simulink model "slam"  (R2018a)
settings: Solver=VariableStepAuto  StartTime=0.0  StopTime=25  RelTol=1e-3
model workspace (MAT data in the model file):
  SL_ROS_VariableLengthArrays_MaxSizes.CommonInfo.ArrayTruncateAction = 'EmitWarning'
  SL_ROS_VariableLengthArrays_MaxSizes.MsgTypeMap = containers.Map
  SL_ROS_VariableLengthArrays_MaxSizes.MsgTypeMap.serialization.keys = {'sensor_msgs/LaserScan'}
  SL_ROS_VariableLengthArrays_MaxSizes.MsgTypeMap.serialization.values{1}(1).PropertyName = 'Intensities'
  SL_ROS_VariableLengthArrays_MaxSizes.MsgTypeMap.serialization.values{1}(1).DataType = 'single'
  SL_ROS_VariableLengthArrays_MaxSizes.MsgTypeMap.serialization.values{1}(1).MaxLength = 360
  SL_ROS_VariableLengthArrays_MaxSizes.MsgTypeMap.serialization.values{1}(2).PropertyName = 'Ranges'
  SL_ROS_VariableLengthArrays_MaxSizes.MsgTypeMap.serialization.values{1}(2).DataType = 'single'
  SL_ROS_VariableLengthArrays_MaxSizes.MsgTypeMap.serialization.values{1}(2).MaxLength = 360
  SL_ROS_VariableLengthArrays_MaxSizes.MsgTypeMap.serialization.uniformity = 0
  SL_ROS_VariableLengthArrays_MaxSizes.MsgTypeMap.serialization.keyType = 'char'
  SL_ROS_VariableLengthArrays_MaxSizes.MsgTypeMap.serialization.valueType = 'any'
undefined symbols (not defined in the file or in its folder): Angular, Linear
libraries: robotlib x6, simulink x1
settings Model: EnablePacing=on  Creator=gabriele  LastModifiedBy=gabriele

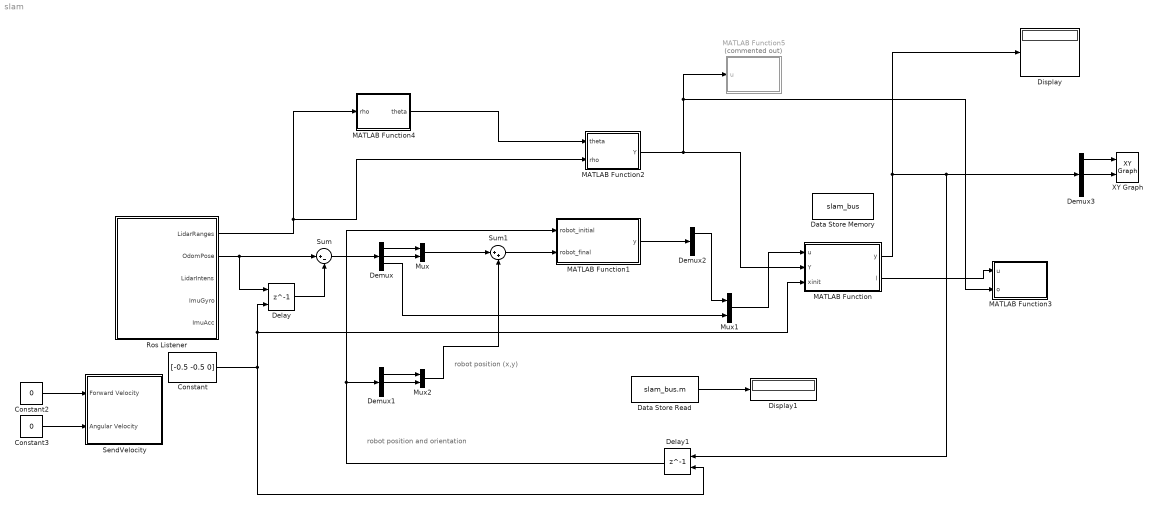
== system slam ==
  note: robot position
      | and orientation
  note: robot position (x,y)
  Constant : Constant  Value=[-0.5 -0.5 0]
  Constant2 : Constant  Value=0
  Constant3 : Constant  Value=0
  Data Store Memory : DataStoreMemory  DataStoreName=slam_bus  ReadBeforeWriteMsg=warning  WriteAfterWriteMsg=warning  WriteAfterReadMsg=warning  ShowAdditionalParam=off  OutDataTypeStr=Bus: slam_bus_t
  Data Store Read : DataStoreRead  DataStoreName=slam_bus  DataStoreElements=slam_bus.m
  Delay : Delay  DelayLength=1  InitialConditionSource=Input port  InitialCondition=[-0.5 -0.5 0]
      settings: InputPortMap=u0,p4
  Delay1 : Delay  DelayLength=1  InitialConditionSource=Input port  InitialCondition=zeros(3,1)
      settings: InputPortMap=u0,p4
  Demux : Demux  Outputs=3
  Demux1 : Demux  Outputs=3
  Demux2 : Demux  Outputs=2
  Demux3 : Demux  Outputs=3
  Display : Display
  Display1 : Display
  MATLAB Function : MATLAB Function  TreatAsAtomicUnit=on  mask{q=[0.1;0.1], s=[0.1;0.1]}
      mask prompts: q "Odometry Gaussian Noise"; s "Lidar Gaussian Noise"
  MATLAB Function1 : MATLAB Function  TreatAsAtomicUnit=on
  MATLAB Function2 : MATLAB Function  TreatAsAtomicUnit=on
  MATLAB Function3 : MATLAB Function  TreatAsAtomicUnit=on
  MATLAB Function4 : MATLAB Function  TreatAsAtomicUnit=on
  MATLAB Function5 : MATLAB Function  Commented=on  TreatAsAtomicUnit=on
  Mux : Mux  Inputs=2
  Mux1 : Mux  Inputs=2
  Mux2 : Mux  Inputs=2
  Ros Listener : Subsystem
  SendVelocity : Subsystem
  Sum : Sum  Inputs=|+-
  Sum1 : Sum  Inputs=|++
  XY Graph : simulink/Sinks/XY Graph  xmin=-1  xmax=1  ymin=-1  ymax=1  st=-1
  wires:
  Demux3/2 -> XY Graph/2
  Sum/1 -> Demux/1
  Ros Listener/2(OdomPose) -> Delay/1, Sum/1
  Delay1/1 -> Demux1/1, MATLAB Function1/1(robot_initial)
  Mux1/1 -> MATLAB Function/1(u)
  Delay/1 -> Sum/2
  MATLAB Function2/1(Y) -> MATLAB Function3/2(o), MATLAB Function5/1(u), MATLAB Function/2(Y)
  Mux/1 -> Sum1/1
  MATLAB Function/1(y) -> Display/1, Delay1/1, Demux3/1
  Demux/2 -> Mux/2
  Demux3/1 -> XY Graph/1
  Demux1/2 -> Mux2/2
  MATLAB Function1/1(y) -> Demux2/1
  Demux/1 -> Mux/1
  Mux2/1 -> Sum1/2
  Sum1/1 -> MATLAB Function1/2(robot_final)
  Demux1/1 -> Mux2/1
  Constant3/1 -> SendVelocity/2(Angular Velocity)
  Constant2/1 -> SendVelocity/1(Forward Velocity)
  Demux/3 -> Mux1/2
  Demux2/1 -> Mux1/1
  Ros Listener/1(LidarRanges) -> MATLAB Function2/2(rho), MATLAB Function4/1(rho)
  MATLAB Function4/1(theta) -> MATLAB Function2/1(theta)
  MATLAB Function/2(l) -> MATLAB Function3/1(u)
  Constant/1 -> Delay1/2, MATLAB Function/3(xinit), Delay/2
  Data Store Read/1 -> Display1/1

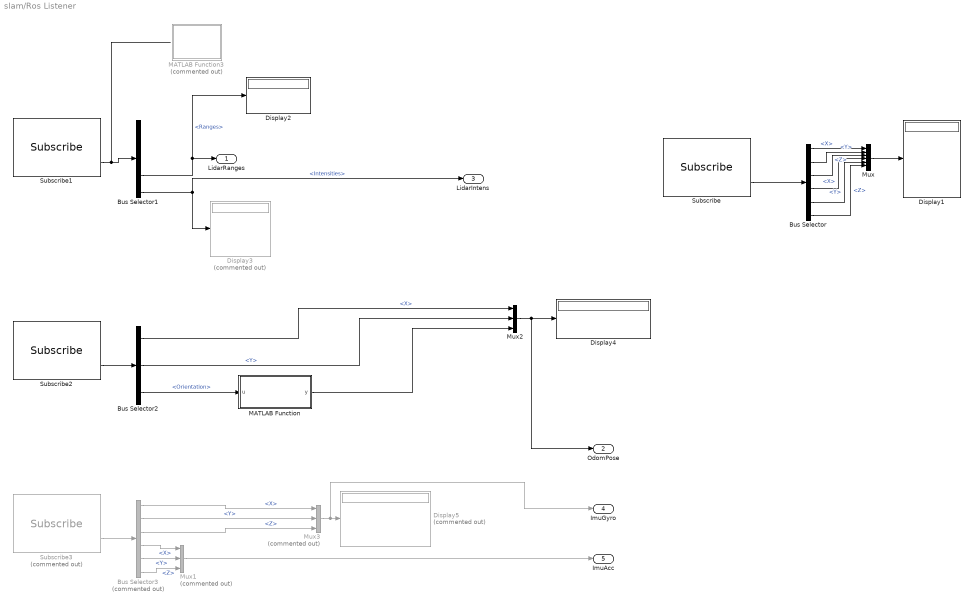
== system slam/Ros Listener ==
  Bus Selector : BusSelector  OutputSignals=Linear.X,Linear.Y,Linear.Z,Angular.X,Angular.Y,Angular.Z
  Bus Selector1 : BusSelector  OutputSignals=AngleMin,AngleMax,AngleIncrement,Ranges,Intensities
  Bus Selector2 : BusSelector  OutputSignals=Pose.Pose.Position.X,Pose.Pose.Position.Y,Pose.Pose.Orientation
  Bus Selector3 : BusSelector  Commented=on  OutputSignals=AngularVelocity.X,AngularVelocity.Y,AngularVelocity.Z,LinearAcceleration.X,LinearAcceleration.Y,LinearAcceleration.Z
  Display1 : Display
  Display2 : Display
  Display3 : Display  Commented=on
  Display4 : Display
  Display5 : Display  Commented=on
  MATLAB Function : MATLAB Function  TreatAsAtomicUnit=on
  MATLAB Function3 : MATLAB Function  Commented=on  TreatAsAtomicUnit=on
  Mux : Mux  Inputs=6
  Mux1 : Mux  Commented=on  Inputs=3
  Mux2 : Mux  Inputs=3
  Mux3 : Mux  Commented=on  Inputs=3
  Subscribe : robotlib/Subscribe  SourceLibraryInfo=This block requires Robotics System Toolbox  topicSource=Select from ROS network  topic=/mobile_base/commands/velocity  messageType=geometry_msgs/Twist  sampleTime=-1  messageQueueLength=1
      settings: SourceProductBaseCode=RO
  Subscribe1 : robotlib/Subscribe  SourceLibraryInfo=This block requires Robotics System Toolbox  topicSource=Select from ROS network  topic=/scan  messageType=sensor_msgs/LaserScan  sampleTime=-1  messageQueueLength=1
      settings: SourceProductBaseCode=RO
  Subscribe2 : robotlib/Subscribe  SourceLibraryInfo=This block requires Robotics System Toolbox  topicSource=Select from ROS network  topic=/odom  messageType=nav_msgs/Odometry  sampleTime=-1  messageQueueLength=1
      settings: SourceProductBaseCode=RO
  Subscribe3 : robotlib/Subscribe  Commented=on  SourceLibraryInfo=This block requires Robotics System Toolbox  topicSource=Specify your own  topic=/imu  messageType=sensor_msgs/Imu  sampleTime=-1  messageQueueLength=1
      settings: SourceProductBaseCode=RO
  LidarRanges : Outport
  OdomPose : Outport  Port=2
  LidarIntens : Outport  Port=3
  ImuGyro : Outport  Port=4
  ImuAcc : Outport  Port=5
  wires:
  Subscribe3/2 -> Bus Selector3/1
  Bus Selector1/4 -> Display2/1, LidarRanges/1  "<Ranges>"
  Bus Selector1/5 -> LidarIntens/1, Display3/1  "<Intensities>"
  Subscribe1/2 -> Bus Selector1/1
  Subscribe2/2 -> Bus Selector2/1
  Bus Selector2/1 -> Mux2/1  "<X>"
  Bus Selector2/2 -> Mux2/2  "<Y>"
  Mux2/1 -> OdomPose/1, Display4/1
  Bus Selector3/4 -> Mux1/1  "<X>"
  Bus Selector3/5 -> Mux1/2  "<Y>"
  Bus Selector3/6 -> Mux1/3  "<Z>"
  Bus Selector3/2 -> Mux3/2  "<Y>"
  Bus Selector3/1 -> Mux3/1  "<X>"
  Bus Selector3/3 -> Mux3/3  "<Z>"
  Mux3/1 -> ImuGyro/1, Display5/1
  Mux1/1 -> ImuAcc/1
  Bus Selector/5 -> Mux/5  "<Y>"
  Bus Selector/2 -> Mux/2  "<Y>"
  Bus Selector/1 -> Mux/1  "<X>"
  Bus Selector/6 -> Mux/6  "<Z>"
  Bus Selector/4 -> Mux/4  "<X>"
  Bus Selector/3 -> Mux/3  "<Z>"
  Mux/1 -> Display1/1
  Subscribe/2 -> Bus Selector/1
  Bus Selector2/3 -> MATLAB Function/1(u)  "<Orientation>"
  MATLAB Function/1(y) -> Mux2/3

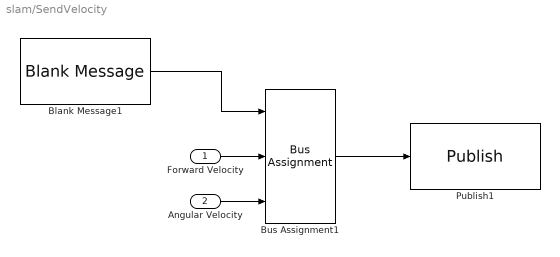
== system slam/SendVelocity ==
  Forward Velocity : Inport
  Angular Velocity : Inport  Port=2
  Blank Message1 : robotlib/Blank Message  SourceLibraryInfo=This block requires Robotics System Toolbox  messageType=geometry_msgs/Twist  SampleTime=-1
      settings: SourceProductBaseCode=RO
  Bus Assignment1 : BusAssignment  AssignedSignals=Linear.X,Angular.Z
  Publish1 : robotlib/Publish  SourceLibraryInfo=This block requires Robotics System Toolbox  topicSource=Select from ROS network  topic=/cmd_vel  messageType=geometry_msgs/Twist  messageQueueLength=5
      settings: SourceProductBaseCode=RO
  wires:
  Blank Message1/1 -> Bus Assignment1/1
  Forward Velocity/1 -> Bus Assignment1/2
  Angular Velocity/1 -> Bus Assignment1/3
  Bus Assignment1/1 -> Publish1/1

== matlab function slam/MATLAB Function1 ==
  data: robot_initial input; y output; robot_final input
function y = fcn(robot_initial, robot_final)

y = toFrame(robot_initial, robot_final);

end

function [pf, PF_f, PF_p] = toFrame(F , p)
% TOFRAME transform point P from global frame to frame F
%
% In:
%   F:      reference frame F = [f x ; f y ; f alpha]
%   p:      point in global frame p = [p x ; p y]
% Out:
%   pf:     point in frame F
%   PF_f:   Jacobian wrt F
%   PF_p:   Jacobian wrt p

% (c) 2010, 2011, 2012 Joan Sola

t = F(1:2);
a = F(3);

R = [cos(a) -sin(a) ; sin(a) cos(a)];

pf = R' * (p - t);

if nargout > 1 % Jacobians requested
    px = p(1);
    py = p(2);
    x = t(1);
    Y = t(2);

    PF_f = [ ...
        [ -cos(a), -sin(a), cos(a)*(py - Y) - sin(a)*(px - x)]
        [ sin(a), -cos(a), - cos(a)*(px - x) - sin(a)*(py - Y)]];
    
    PF_p = R';
end
end

== matlab function slam/MATLAB Function ==
  data: u input; Y input; y output; slam_bus data_store_memory; q parameter; s parameter; l output; xinit input
function [y, l] = fcn(u, Y, q, s, xinit)

global slam_bus;

r = [1 2 3];

slam_bus_copy = slam_bus;

if ~slam_bus_copy.first
    slam_bus_copy.x(r) = xinit;
    slam_bus_copy.first = true;
end

idx = randperm(length(Y));
% idx = idx(randperm(length(idx)));
Y = Y(:, idx);

slam_bus = ekf_slam(slam_bus_copy, u, Y, s, q);

y = slam_bus.x(r);
l = slam_bus.x(4:end);

fprintf("The numer of landmarks is %f.\n", slam_bus.m);

end

function slam_bus = ekf_slam(slam_bus, u, Y, s, q)

x           = slam_bus.x;
P           = slam_bus.P;
m           = slam_bus.m;
landcounter = slam_bus.landcounter;

% N = size(x, 2) - 3;
N = 32;

S = diag(s.^2);
r = [1 2 3];

%% FUNCTION START
[x,P] = slam2d_move_estimator(x,P,u,m,q);

% For each point, calculate its closes landmark with Mahalanolis distance,
% then if the distance is under a certain treshold update said landmark
% (then skip said landmark in the future)

np = size(Y, 2); % Number of points

landmarks_corrected = false(1, m);
points_used = false(1, np);

% Indexes of all active landmarks in x
ll = 3+1 : 3 + m*2;

% a. create dynamic map pointers to be used hereafter
rm = [r, ll];	% all used states: robot and landmarks

% accepted = false;

z       = zeros(2, m, np);
Z       = zeros(2, 2, m, np);
E_rl    = zeros(2, 5, m, np);
dist    = inf(m, np);

% For each point
for j = 1:np
    
    % For each landmark
    for i = 1:m
        Yj = Y(:, j);
        
        %landmark_index = i;
        l = landmark_i(i);
        
        rl	= [r, l'];               % pointers to robot and lmk.
        
        % Compute E matrix
        [ei, E_r_ij, E_l_ij] = observe(x(r), x(l));  % this is h(x) in EKF
        E_rl_ij	= [E_r_ij , E_l_ij];          % expectation Jacobian
        E_ij	= E_rl_ij * P(rl, rl) * E_rl_ij';
        
        % innovation: Gaussian {z,Z}
        z_ij = Yj - ei; % this is z = y - h(x) in EKF
        % we need values around zero for angles:
        if z_ij(2) > pi
            z_ij(2) = z_ij(2) - 2*pi;
        end
        if z_ij(2) < -pi
            z_ij(2) = z_ij(2) + 2*pi;
        end
        Z_ij = S + E_ij;
        
        dist(i, j) = z_ij' * Z_ij^-1 * z_ij;
        z(:, i, j) = z_ij;
        Z(:, :, i, j) = Z_ij;
        E_rl(:, :, i, j) = E_rl_ij;
    end
end

% Now that I calculated all the distances and matrices, I can use the least
% one for each landmark to update it

for i = 1:m
    % This check does not check wether a point as already been used or not
    [distmin, j] = min(dist(i, :));
    
    % This landmark will be updated only if there is a sufficiently near
    % point to update it
    
    % Individual compatibility check at Mahalanobis distance of 3-sigma
    % (See appendix of documentation file 'SLAM course.pdf')
    if ~isempty(distmin) && distmin < 4 % 9
        
        l = landmark_i(i);
        
        rl	= [r , l'];              % pointers to robot and lmk.
        
        % Compute E matrix
        [ei, E_r_ij, E_l_ij] = observe(x(r), x(l));  % this is h(x) in EKF
        
        E_rl_ij          = [E_r_ij , E_l_ij];          % expectation Jacobian
        E_ij             = E_rl_ij * P(rl, rl) * E_rl_ij';
        
        % innovation: Gaussian {z,Z}
        z_ij = Y(:, j) - ei; % this is z = y - h(x) in EKF
        
        % we need values around zero for angles:
        if z_ij(2) > pi
            z_ij(2) = z_ij(2) - 2*pi;
        end
        if z_ij(2) < -pi
            z_ij(2) = z_ij(2) + 2*pi;
        end
        Z_ij = S + E_ij;
        
        % Kalman gain
        K = P(rm, rl) * E_rl_ij' * Z_ij^-1; % this is K = P*H'*Z^-1 in EKF
        % map update (use pointer rm)
        
        x(rm)    = x(rm)    + K*z_ij;
        P(rm,rm) = P(rm,rm) - K*Z_ij*K';
        
        landmarks_corrected(i) = true;
        points_used(j) = true;
    end
    
    % Else skip landmark
end

% Now I need to pick one of remaining points and check wether I should add
% it to the set of landmarks

% remaining_points_idx = find(~points_used);
%
% mindistances = inf(1, length(remaining_points_idx));
%
% if num_landmarks > 0
%     for idx = 1:length(remaining_points_idx)
%        j = remaining_points_idx(idx);
%        mindistances(idx) = min(dist(:, j));
%     end
%
%     [distmin,maxidx] = max(mindistances(idx));
% else
%     distmin = inf;
%     maxidx = 1;
% end
%
% % Consider using euclidean distance instead of Maholanian one
% if ~isempty(distmin) && num_landmarks < 32 && distmin > 40
%     j = remaining_points_idx(maxidx);
%     Y_NEW = Y(:, j);
%     accepted = true;
% end

%% TODO: ADD PARAMETER FOR NUMBER OF ACCEPTED POINTS
%% TODO: CHANGE ITERATION ON REMAINING_POINTS_IDX

remaining_points_idx = find(~points_used);
accepted = 0;
while accepted < 1 && ~isempty(remaining_points_idx) && m < N
    j = remaining_points_idx(1);
    
    if isempty(dist)
        distmin = inf;
    else
        distmin = min(dist(:, j));
    end
    
    
    if isempty(distmin) || distmin > 40
        Yj = Y(:, j);
        accepted = accepted+1;
        
        % Should add a new point to the landmarks set, only if its Mahalonis
        % distance with respect to previous points is greater than a certain
        % treshold
        
        m = m+1;
        
        l = landmark_i(m);
        
        landcounter(m) = 2;
        
        % initialization
        [x(l), L_r, L_y] = invObserve(x(r), Yj);
        P(l,rm)          = L_r * P(r,rm);
        P(rm,l)          = P(l,rm)';
        P(l,l)           = L_r * P(r,r) * L_r' + L_y * S * L_y';
    end
    
    remaining_points_idx(1) = [];
end

landcounter(landmarks_corrected) = landcounter(landmarks_corrected) + 1;
landcounter(~landmarks_corrected) = landcounter(~landmarks_corrected) - 0.5;

%% TODO: CHANGE TO A PARAMETER
landcounter(landcounter > 2) = 2;

%% TODO: CHANGE REMOVAL

remove_these = find(landcounter < 0); % <= ?
remove_these(4:end) = [];

Nremove = numel(remove_these);

if Nremove > 0
    new_order   = 1:N;
    
    other_rows = 1:N;
    other_rows = other_rows(~ismember(other_rows, remove_these));
    
    for i = 1:N
        if i <= N-Nremove
            new_order(i) = other_rows(i);
        else
            new_order(i) = remove_these(N-i+1);
        end
    end
    % new_order = [other_rows remove_these];
    
    x_new_order = [r zeros(1, N*2)];
    for i = 1:N
        l = landmark_i(i);
        newl = landmark_i(new_order(i));
        x_new_order(l) = newl;
    end
    
    x           = x(x_new_order, :);
    P           = P(x_new_order, x_new_order);
    
    landcounter  = landcounter(:, new_order); %% TODO: CHECK
    
    % Then I need to set to zero last rows and columns
    N_remove = numel(remove_these);
    remove_indexes = N-N_remove+1: N;
    x_remove_indexes = N*2+3 - (N_remove*2) +1 : N*2+3 ;
    
    
    x(x_remove_indexes, :) = 0;
    P(x_remove_indexes, :) = 0;
    P(:, x_remove_indexes) = 0;
    
    landcounter(remove_indexes) = 0;
    
    m = m-N_remove;
end


%% FUNCTION END



slam_bus.x              = x;
slam_bus.P              = P;
slam_bus.m              = m;
slam_bus.landcounter    = landcounter;

end

function [x,P] = slam2d_move_estimator(x,P,u,m,q)

Q = diag(q.^2);     % covariances matrix
r = [1 2 3];

if m > 0
    ll = 3 + 2*m;
    ll = 3+1 : ll;
    ll = reshape(ll', 1, numel(ll));
else
    ll = [];
end

% b. Prediction -- robot motion
[x(r), R_r, R_n] = move(x(r), u, zeros(2,1));	% Estimator perturbed with n

P(r,ll) = R_r * P(r,ll);                        % See PDF notes 'SLAM course.pdf'
P(ll,r) = P(r,ll)';
P(r,r)  = R_r * P(r,r) * R_r' + R_n * Q * R_n';

end

function l = landmark_i(i)
    l = 3 + 2*(i-1);
    l = [
        l+1;
        l+2
        ];
end

function [pw, PW_f, PW_pf] = fromFrame(F, pf)
% FROMFRAME Transform a point PF from local frame F to the global frame.
%
% In:
%   F:      reference frame F = [f x ; f y ; f alpha]
%   pf:     point in frame F pf = [pf x ; pf y]
% Out:
%   pw:     point in global frame
%   PW_f:   Jacobian wrt F
%   PW_pf:  Jacobian wrt pf

% (c) 2010, 2011, 2012 Joan Sola

t = F(1:2);
a = F(3);

R = [cos(a) -sin(a) ; sin(a) cos(a)];
pw = R*pf + repmat(t,1,size(pf,2)); % Allow for multiple points

if nargout > 1 % Jacobians requested
    px = pf(1);
    py = pf(2);
    PW_f = [...
        [ 1, 0, - py*cos(a) - px*sin(a)]
        [ 0, 1,   px*cos(a) - py*sin(a)]];
    PW_pf = R;
end
end

function [p, P_y] = invScan(y)
% INVSCAN Backproject a range?and?bearing measure into a 2D point.
%
% In:
%   y:      range-and-bearing measurement y = [range ; bearing]
% Out:
%   p:      point in sensor frame p = [p_x ; p_y]
%   P_y:    Jacobian wrt y

% (c) 2010, 2011, 2012 Joan Sola

d = y(1);
a = y(2);
px = d*cos(a);
py = d*sin(a);

p = [px;py];

if nargout > 1 % Jacobians requested
    P_y = [...
        cos(a) , -d*sin(a)
        sin(a) , d*cos(a)];
end
end

function [y, Y_p] = scan (p)
% SCAN perform a range-and-bearing measure of a 2D point.
%
% In:
%   p:      point in sensor frame p = [p_x ; p_y]
% Out:
%   y:      measurement y = [range ; bearing]
%   Y_p:    Jacobian wrt p

% (c) 2010, 2011, 2012 Joan Sola
px = p(1);
py = p(2);
d = sqrt(px^2+py^2);
a = atan2(py,px);
% a = atan(py/px); % use this line if you are in symbolic mode.
y = [d;a];
if nargout > 1 % Jacobians requested
    Y_p = [...
        px/sqrt(px^2+py^2) , py/sqrt(px^2+py^2)
        -py/(px^2*(py^2/px^2 + 1)), 1/(px*(py^2/px^2 + 1)) ];
end
end

function [pf, PF_f, PF_p] = toFrame(F , p)
% TOFRAME transform point P from global frame to frame F
%
% In:
%   F:      reference frame F = [f x ; f y ; f alpha]
%   p:      point in global frame p = [p x ; p y]
% Out:
%   pf:     point in frame F
%   PF_f:   Jacobian wrt F
%   PF_p:   Jacobian wrt p

% (c) 2010, 2011, 2012 Joan Sola

t = F(1:2);
a = F(3);

R = [cos(a) -sin(a) ; sin(a) cos(a)];

pf = R' * (p - t);

if nargout > 1 % Jacobians requested
    px = p(1);
    py = p(2);
    x = t(1);
    Y = t(2);

    PF_f = [ ...
        [ -cos(a), -sin(a), cos(a)*(py - Y) - sin(a)*(px - x)]
        [ sin(a), -cos(a), - cos(a)*(px - x) - sin(a)*(py - Y)]];
    
    PF_p = R';
end
end

function [dist,closest_i] = closest(vec,mat)
%CLOSEST Determines the index of closest vector to the one provided in
%input as range-and-bearing coordinates
%   Vectors are stored as columns

r = 1;
b = 2;

[~,m] = size(mat);

if m == 0
    closest_i = 0;
    dist = inf;
    return;
end

distances = zeros(1,m);

for i = 1:m
    % Polar distance
    distances(i) = vec(r)^2 + mat(r,i)^2 - 2 * vec(r) * mat(r,i) * cos(vec(b) - mat(b,i));
end

[dist, closest_i] = min(distances);

dist = sqrt(dist);

end

function [p, P_r, P_y] = invObserve(r, y)
% INVOBSERVE Backproject a range-and-bearing measurement and transform
% to map frame.
%
% In:
%   r:      robot frame     r = [r x ; r y ; r alpha]
%   y:      measurement     y = [range ; bearing]
% Out:
%   p:      point in sensor frame
%   P_r:    Jacobian wrt r
%   P_y:    Jacobian wrt y

% (c) 2010, 2011, 2012 Joan Sola

if nargout == 1 % No Jacobians requested
    p = fromFrame(r, invScan(y));
else % Jacobians requested
    [p_r, PR_y] = invScan(y);
    [p, P_r, P_pr] = fromFrame(r, p_r);
    % here the chain rule !
    P_y = P_pr * PR_y;
end
end


function [ro, RO_r, RO_n] = move(r, u, n)
% MOVE Robot motion, with separated control and perturbation inputs.
%
% In:
%   r:      robot pose      r = [x ; y ; alpha]
%   u:      control signal  u = [d_x ; d_alpha]
%   n:      perturbation, additive to control signal
% Out:
%   ro:     updated robot pose
%   RO_r:   Jacobian d(ro) / d(r)
%   RO_n:   Jacobian d(ro) / d(n)

% (c) 2010, 2011, 2012 Joan Sola

a = r(3);
dx = u(1) + n(1);
da = u(2) + n(2);

ao = a + da;

if ao > pi
    ao = ao - 2*pi;
end
if ao < -pi
    ao = ao + 2*pi;
end

% build position increment dp=[dx;dy], from control signal dx
dp = [dx;0];

if nargout == 1 % No Jacobians requested
    to = fromFrame(r, dp);
else % Jacobians requested
    [to, TO_r, TO_dt] = fromFrame(r, dp);
    AO_a = 1;
    AO_da = 1;
    
    RO_r = [TO_r ; 0 0 AO_a];
    RO_n = [TO_dt(:,1) zeros(2,1) ; 0 AO_da];
end

ro = [to;ao];
end

function [y, Y_r, Y_p] = observe(r, p)
% OBSERVE Transform a point P to robot frame and take a
% range-and-bearing measurement.
%
% In:
%   r:      robot frame r = [r x ; r y ; r alpha]
%   p:      point in global frame p = [p x ; p y]
% Out:
%   y:      range-and-bearing measurement
%   Y_r:    Jacobian wrt r
%   Y_p:    Jacobian wrt p

% (c) 2010, 2011, 2012 Joan Sola
if nargout == 1 % No Jacobians requested
    y = scan(toFrame(r,p));
else % Jacobians requested
    [pr, PR_r, PR_p] = toFrame(r, p);
    [y, Y_pr] = scan(pr);
    
    % The chain rule!
    Y_r = Y_pr * PR_r;
    Y_p = Y_pr * PR_p;
end
end

== matlab function slam/Ros Listener/MATLAB Function ==
  data: u input; y output
function y = Orientation2Yaw(u)

x = quat2eul([u.W u.X u.Y u.Z]);
y = x(1);

== matlab function slam/MATLAB Function2 ==
  data: theta input; Y output; rho input
function Y = fcn(theta, rho)

Y = [rho'; theta'];

== matlab function slam/MATLAB Function3 ==
  data: u input; o input
function fcn(u, o)

m = numel(u)/2;

lids = 3+1:3+m*2;
idxx = mod(lids,2);

idx = find(~idxx);
idy = find(idxx);

lx   = u(idx); % all x-coordinates
ly   = u(idy); % all y-coordinates

% lx(lx==0 && ly==0) = [];
% ly(lx==0 && ly==0) = [];

x = zeros(1, length(o));
y = x;

for i = 1:length(u)
    x(i) = o(1, i) * cos(o(2, i));
    y(i) = o(1, i) * sin(o(2, i));
end

plot(lx,ly, '.b', x, y, '+r');
xlim([-8 8]);
ylim([-8 8]);

drawnow;

end

== matlab function slam/Ros Listener/MATLAB Function3 ==
function fcn()

scansub = rossubscriber('/scan');
scan = receive(scansub);

cartScanData = scan.readCartesian;
cartScanData(:,3) = 0;
homScanData = cart2hom(cartScanData);

[angles,ranges] = cart2pol(homScanData(:,1),...
                           homScanData(:,2));
                       
[x,y] = pol2cart(angles,ranges);

coder.extrinsic('plot');
plot(x,y, '.');
xlim([-5,5]);
ylim([-5,5]);


% theta = 0:127;
% 
% %theta = 0:pi*2/127:pi*2;
% % fprintf("The size of theta is %f, while size of rho is %f.\n", length(theta), length(rho));
% 
% [x,y] = pol2cart(theta' * pi * 2 / 127, rho);
% 

%[x,y] = pol2cart(theta,rho);

== matlab function slam/MATLAB Function4 ==
  data: rho input; theta output
function theta = fcn(rho)
N = length(rho);
theta = (0:N-1)';
theta = theta * pi * 2 / N;

== matlab function slam/MATLAB Function5 ==
  data: u input
function fcn(u)

x = zeros(1, length(u));
y = x;

for i = 1:length(u)
    x(i) = u(1, i) * cos(u(2, i));
    y(i) = u(1, i) * sin(u(2, i));
end

%plot(x,y, 'r.');
%drawnow;

end
